simulink library "VehicleSimulation"  (R2014a)
settings: Solver=ode45  SolverMode=SingleTasking  StartTime=0.0  StopTime=10.0  RelTol=1e-3
undefined symbols (not defined in the file): bs, eff, fs, gpsins, gr, Js, kM, ljt, lma, param, rjt, rma, sglu, sr
libraries: simulink x2, VehicleSimulation x1
(part 2 of 2)

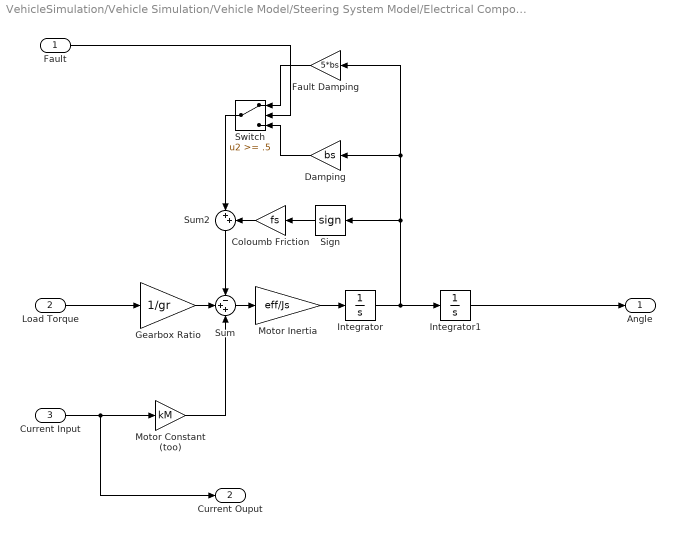
== system VehicleSimulation/Vehicle Simulation/Vehicle Model/Steering System Model/Electrical Components and Motors/Motors/Left Motor ==
  Fault : Inport
  Load Torque : Inport  Port=2
  Current Input : Inport  Port=3
  Coloumb Friction : Gain  Gain=fs  SaturateOnIntegerOverflow=on  OutDataTypeStr=Inherit: Same as input  ParamDataTypeStr=Inherit: Same as input
  Damping : Gain  Gain=bs  SaturateOnIntegerOverflow=on  OutDataTypeStr=Inherit: Same as input  ParamDataTypeStr=Inherit: Same as input
  Fault Damping : Gain  Gain=5*bs  SaturateOnIntegerOverflow=on  OutDataTypeStr=Inherit: Same as input  ParamDataTypeStr=Inherit: Same as input
  Gearbox Ratio : Gain  Gain=1/gr  SaturateOnIntegerOverflow=on  OutDataTypeStr=Inherit: Same as input  ParamDataTypeStr=Inherit: Same as input
  Integrator : Integrator
  Integrator1 : Integrator
  Motor Constant (too) : Gain  Gain=kM  SaturateOnIntegerOverflow=on  OutDataTypeStr=Inherit: Same as input  ParamDataTypeStr=Inherit: Same as input
  Motor Inertia : Gain  Gain=eff/Js  SaturateOnIntegerOverflow=on  OutDataTypeStr=Inherit: Same as input  ParamDataTypeStr=Inherit: Same as input
  Sign : Signum  ZeroCross=off
  Sum : Sum  Inputs=-++  SaturateOnIntegerOverflow=on
  Sum2 : Sum  Inputs=|++  SaturateOnIntegerOverflow=on
  Switch : Switch  Threshold=.5  ZeroCross=off  SaturateOnIntegerOverflow=on
  Angle : Outport
  Current Ouput : Outport  Port=2
  wires:
  Current Input/1 -> Motor Constant (too)/1, Current Ouput/1
  Load Torque/1 -> Gearbox Ratio/1
  Motor Constant (too)/1 -> Sum/3
  Switch/1 -> Sum2/1
  Sum2/1 -> Sum/1
  Coloumb Friction/1 -> Sum2/2
  Sign/1 -> Coloumb Friction/1
  Gearbox Ratio/1 -> Sum/2
  Integrator1/1 -> Angle/1
  Integrator/1 -> Integrator1/1, Sign/1, Fault Damping/1, Damping/1
  Motor Inertia/1 -> Integrator/1
  Sum/1 -> Motor Inertia/1
  Damping/1 -> Switch/3
  Fault Damping/1 -> Switch/1
  Fault/1 -> Switch/2

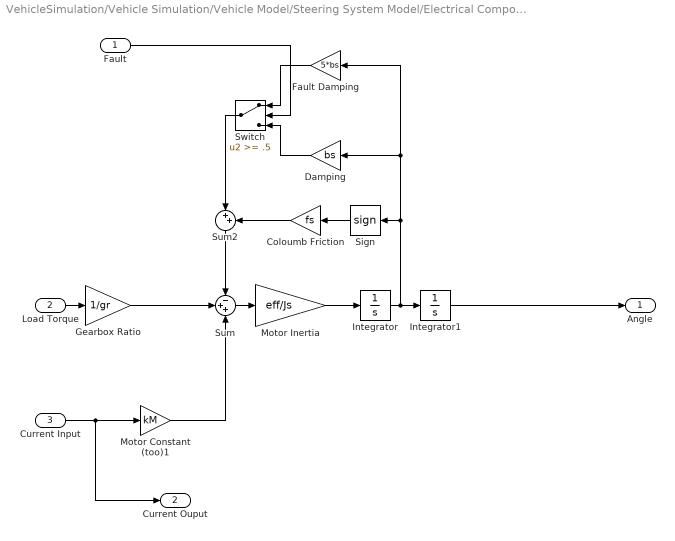
== system VehicleSimulation/Vehicle Simulation/Vehicle Model/Steering System Model/Electrical Components and Motors/Motors/Right Motor ==
  Fault : Inport
  Load Torque : Inport  Port=2
  Current Input : Inport  Port=3
  Coloumb Friction : Gain  Gain=fs  SaturateOnIntegerOverflow=on  OutDataTypeStr=Inherit: Same as input  ParamDataTypeStr=Inherit: Same as input
  Damping : Gain  Gain=bs  SaturateOnIntegerOverflow=on  OutDataTypeStr=Inherit: Same as input  ParamDataTypeStr=Inherit: Same as input
  Fault Damping : Gain  Gain=5*bs  SaturateOnIntegerOverflow=on  OutDataTypeStr=Inherit: Same as input  ParamDataTypeStr=Inherit: Same as input
  Gearbox Ratio : Gain  Gain=1/gr  SaturateOnIntegerOverflow=on  OutDataTypeStr=Inherit: Same as input  ParamDataTypeStr=Inherit: Same as input
  Integrator : Integrator
  Integrator1 : Integrator
  Motor Constant (too)1 : Gain  Gain=kM  SaturateOnIntegerOverflow=on  OutDataTypeStr=Inherit: Same as input  ParamDataTypeStr=Inherit: Same as input
  Motor Inertia : Gain  Gain=eff/Js  SaturateOnIntegerOverflow=on  OutDataTypeStr=Inherit: Same as input  ParamDataTypeStr=Inherit: Same as input
  Sign : Signum  ZeroCross=off
  Sum : Sum  Inputs=-++  SaturateOnIntegerOverflow=on
  Sum2 : Sum  Inputs=|++  SaturateOnIntegerOverflow=on
  Switch : Switch  Threshold=.5  ZeroCross=off  SaturateOnIntegerOverflow=on
  Angle : Outport
  Current Ouput : Outport  Port=2
  wires:
  Gearbox Ratio/1 -> Sum/2
  Coloumb Friction/1 -> Sum2/2
  Switch/1 -> Sum2/1
  Current Input/1 -> Current Ouput/1, Motor Constant (too)1/1
  Motor Constant (too)1/1 -> Sum/3
  Fault/1 -> Switch/2
  Fault Damping/1 -> Switch/1
  Damping/1 -> Switch/3
  Sum/1 -> Motor Inertia/1
  Motor Inertia/1 -> Integrator/1
  Integrator/1 -> Integrator1/1, Fault Damping/1, Damping/1, Sign/1
  Integrator1/1 -> Angle/1
  Sign/1 -> Coloumb Friction/1
  Sum2/1 -> Sum/1
  Load Torque/1 -> Gearbox Ratio/1
